simulink model "vkr_ch2_tx"  (R2025b)
settings: Solver=FixedStepDiscrete  StartTime=0.0  StopTime=Nsym/Rs  FixedStep=1/Fs_tx  RelTol=1e-3
values from neighbouring files (symbols this model uses):
  k_bits = log2(M)    [compare_all_architectures.m]    (also in compare_round_period_ber.m; compare_sync_direct.m; params_tx.m; run_ber_curve.m)
  Nsym = 10000    [params_tx.m]    (also in run_dynamics.m = 2000; run_sco_test.m = 30000; test_modelsim_io.m = 5000; test_rice_loop.m = 5000)
  rolloff = 0.35    [compare_all_architectures.m]    (also in compare_round_period_ber.m; compare_sync_direct.m; params_tx.m; process_real_data.m = 0.2)
  Rs = 1e6    (= 1000000)    [params_tx.m]    (also in test_sync_loop.m)
  sps_tx = 40    [compare_all_architectures.m]    (also in compare_round_period_ber.m; compare_sync_direct.m = 8; params_tx.m = 8; run_ber_curve.m = 8)
libraries: commrandsrc3 x1, commdigbbndpm3 x1, commfilt2 x1
settings Model: Creator=Gostie2k  LastModifiedBy=Gostie2k

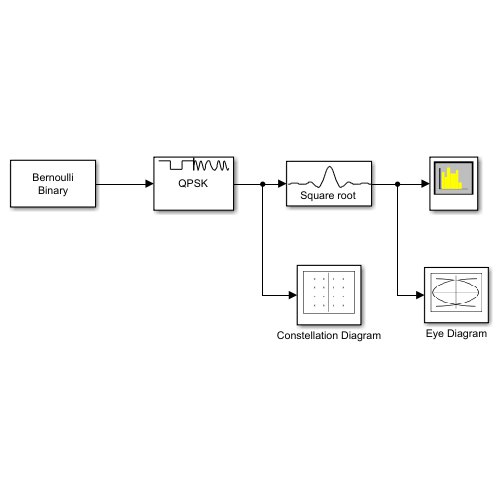
[thumbnail: Simulink's stored preview of the top-level diagram]
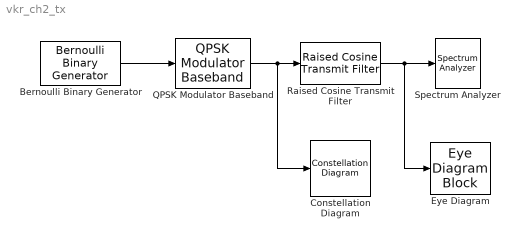
== system vkr_ch2_tx ==
  Bernoulli Binary Generator : commrandsrc3/Bernoulli Binary Generator  ProbabilityOfZero=0.5  SeedSource=Parameter  Seed=12345  SampleTime=1/(Rs*k_bits)  SamplesPerFrame=k_bits*Nsym  OutputDataType=double  SimulateUsing=Interpreted execution
  Constellation Diagram : ConstellationDiagram  WindowPosition=[724.000000,274.000000,600.000000,605.000000,]  ScopeFrameLocation=window  ShowLegend=on  MaximizeAxes=off
  Eye Diagram : EyeDiagramBlock  WindowPosition=[169.000000,14.000000,800.000000,500.000000,]  ScopeFrameLocation=window
  QPSK Modulator Baseband : commdigbbndpm3/QPSK Modulator Baseband  InType=Bit  Enc=Gray  Ph=pi/4  outDtype=double  outWordLen=16  outUDDataType=sfix(16)  outFracLenMode=Best precision  outFracLen=15  outDataTypeStr=double  outLastDataTypeStr=double
  Raised Cosine Transmit Filter : commfilt2/Raised Cosine Transmit Filter  filtType=Square root  R=rolloff  filtSpan=span  N=sps_tx  filterGain=sqrt(sps_tx)  InputProcessing=Columns as channels (frame based)  RateOptions=Enforce single-rate processing  framing=Mute  checkCoeff=off  variableName=rcTxFilt  checkGain=Normalized  sampMode=Mute  saveAsFlag=0  currentFiltSpan=10  D=(10)/2  launchFVT=on  roundingMode=Floor  overflowMode=off  coeffDataTypeStr=Inherit: Same word length as input  coeffMin=[]  coeffMax=[]  coeffLastDataTypeStr=Inherit: Same word length as input  outputDataTypeStr=Inherit: Same as accumulator  outputMin=[]  outputMax=[]  outputLastDataTypeStr=Inherit: Same as accumulator
  Spectrum Analyzer : SpectrumAnalyzer  WindowPosition=[556.000000,483.000000,1018.000000,483.000000,]  ScopeFrameLocation=window  SampleRateSource=Property  SampleRate=Fs_tx  WindowInvariantSamplesPerUpdate=on  Span=8000000  StartFrequency=-4000000  StopFrequency=4000000  YLimits=[-84.9937 20.7573]
  wires:
  Bernoulli Binary Generator/1 -> QPSK Modulator Baseband/1
  QPSK Modulator Baseband/1 -> Constellation Diagram/1, Raised Cosine Transmit Filter/1
  Raised Cosine Transmit Filter/1 -> Eye Diagram/1, Spectrum Analyzer/1
